simulink model "emr_library_custom"  (R2025b)
settings: Solver=ode45  StartTime=0.0  StopTime=10.0  RelTol=1e-3  EnableMultiTasking=on
settings Model: ExtModeTrigMode=oneshot  ExtModeArmWhenConnect=off  Creator=Tony  LastModifiedBy=opatiny
settings SolverCC: AlgebraicLoopSolver=TrustRegion
settings DataIOCC: SaveFormat=Array  SignalLoggingSaveFormat=ModelDataLogs  ReturnWorkspaceOutputs=off  SignalLoggingName=sigsOut
settings OptimizationCC: BooleanDataType=off  ExpressionDepthLimit=2147483647.0  LifeSpan=inf
settings DebuggingCC: SaveWithParameterizedLinksMsg=none  UnderspecifiedInitializationDetection=Classic  MergeDetectMultiDrivingBlocksExec=none  SignalResolutionControl=TryResolveAllWithWarning  MultiTaskDSMMsg=warning  MultiTaskCondExecSysMsg=none  FcnCallInpInsideContextMsg=warning  UnconnectedInputMsg=warning  UnconnectedOutputMsg=warning  UnconnectedLineMsg=warning  StateNameClashWarn=warning  SFUnexpectedBacktrackingDiag=warning  SFNoUnconditionalDefaultTransitionDiag=warning  SFExecutionAtInitializationDiag=none  ArithmeticOperatorsInVariantConditions=warning
settings HardwareCC: ProdBitPerPointer=32.0  ProdBitPerSizeT=32.0  ProdBitPerPtrDiffT=32.0  ProdLargestAtomicFloat=None  ProdIntDivRoundTo=Undefined  ProdEndianess=Unspecified  ProdWordSize=32.0  ProdHWDeviceType=32-bit Generic  TargetUnknown=on
settings ModelReferenceCC: PropagateSignalLabelsOutOfModel=off
settings SFSimCC: SimUseLocalCustomCode=off  CustomCodeUndefinedFunction=UseInterfaceOnly
settings RTWCC: RTWUseLocalCustomCode=off  GPUComputeCapability=3.5
settings CodeAppCC: StateflowObjectComments=on
settings GRTTargetCC: TargetLangStandard=C89/C90 (ANSI)  CombineOutputUpdateFcns=off  GRTInterface=on
settings ConfigComp: CovMetricSettings=dw  CovSaveCumulativeToWorkspaceVar=on  CovSaveSingleToWorkspaceVar=on  CovExternalEMLEnable=off  CovSFcnEnable=off

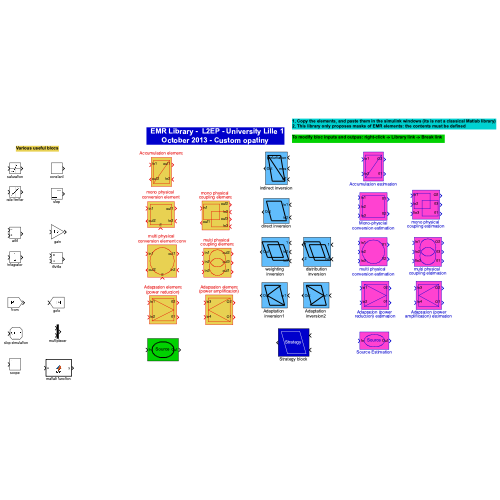
[thumbnail: Simulink's stored preview of the top-level diagram]
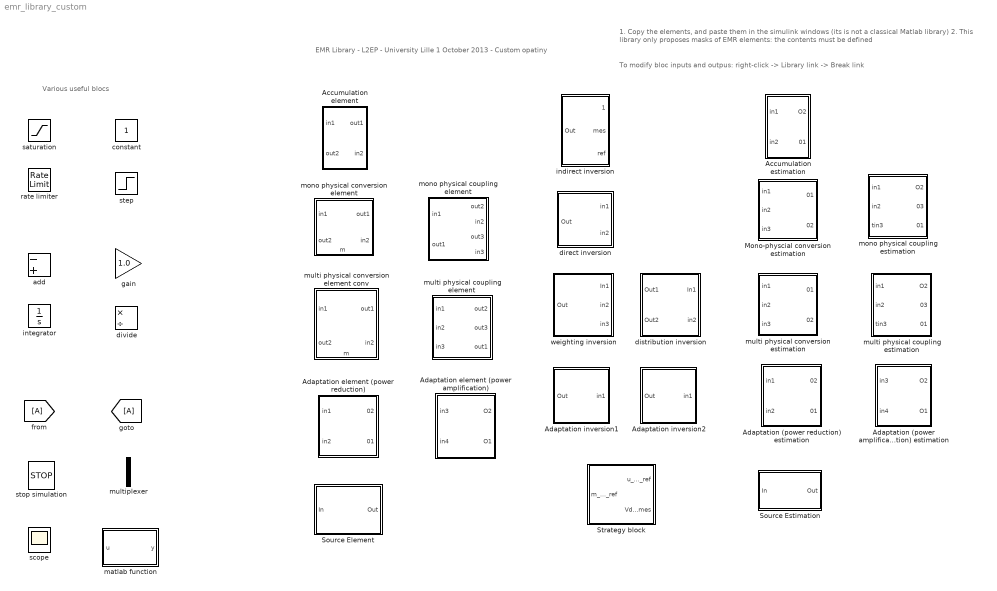
== system emr_library_custom ==
  note: EMR Library -  L2EP - University Lille 1
      | October 2013 - Custom opatiny
  note: 1. Copy the elements, and paste them in the simulink windows (its is not a classical Matlab library)
      | 2. This library only proposes masks of EMR elements: the contents must be defined
  note: Various useful blocs
  note: To modify bloc inputs and outpus: right-click -> Library link -> Break link
  Accumulation element : Subsystem  mask(CM){}
      settings: PortSchema="{\"entries\":[{\"content\":{\"sides\":[{\"content\":{\"connectorIds\":[\"In1\",\"Out2\"]},\"type\":\"ConnectorPlacement.EquallySpacedRectSide\",\"uuid\":\"ce6d3bac-983c-4cc2-8cf0-29bd76c88970\"},{\"content\":{\"connectorIds\":[\"Out1\",\"In2\"],\"side\":\"RIGHT\"},\"type\":\"ConnectorPlacement.EquallySpacedRectSide\",\"uuid\":\"5515666e-487b-4d04-97a1-137c298a6b81\"},{\"content\":{\"side\":\"TOP\"},\"type\":\"ConnectorPlacement.EquallySpacedRectSide\",\"uuid\":\"e218289f-4799-4b6c-b17f-c7c3909bc728\"}]},\"type\":\"ConnectorPlacement.EquallySpacedConnector\",\"uuid\":\"8de20a8e-e66a-466f-89a2-5b2e75b7ec3a\"}],\"packageUris\":[\"http://schema.mathworks.com/mf0/Connector/R2020b\"],\"version\":\"1.0\"}"
      mask Display: plot(0,0,100,100,[10,10,90,90,10],[90,10,10,90,90], [10,90],[10,90])
  Accumulation estimation : Subsystem  AncestorBlock=simulink/REM/EA  mask(CM){}
      mask Display: plot(0,0,100,100,[10,10,90,90,10],[90,10,10,90,90], [10,90],[10,90])
  Adaptation inversion1 : Subsystem  AncestorBlock=simulink/SMC/Inversion EC avec mesure
      mask Display: plot(0,0,100,100, [10,30,90,70,10],[90,10,10,90,90], [90,20,75],[10,50,90])
  Adaptation inversion2 : Subsystem  AncestorBlock=simulink/SMC/Inversion EC avec mesure
      mask Display: plot(0,0,100,100, [10,30,90,70,10],[90,10,10,90,90], [25,80,10],[10,50,90])
  Adaptation (power amplification) estimation : Subsystem  AncestorBlock=simulink/REM/EA  mask(CM){}
      mask Display: plot(0,0,100,100, [10,10,90,90,10],[90,10,10,90,90], [90,10,90],[10,50,90])
  Adaptation (power reduction) estimation : Subsystem  AncestorBlock=simulink/REM/EA  mask(CM){}
      mask Display: plot(0,0,100,100, [10,10,90,90,10],[90,10,10,90,90], [10,90,10],[10,50,90])
  Adaptation element (power amplification) : Subsystem  AncestorBlock=simulink/REM/EA  mask(CM){}
      mask Display: plot(0,0,100,100, [10,10,90,90,10],[90,10,10,90,90], [90,10,90],[10,50,90])
  Adaptation element (power reduction) : Subsystem  mask(CM){}
      mask Display: plot(0,0,100,100, [10,10,90,90,10],[90,10,10,90,90], [10,90,10],[10,50,90])
  Mono-physcial conversion estimation : Subsystem  AncestorBlock=simulink/REM/EC Elec  mask(Hacheur){}
      mask Display: plot(0,0,100,100,[10,10,90,90,10],[90,10,10,90,90])
  Source Element : Subsystem  AncestorBlock=simulink/REM/SE
      mask Display:
      | plot(0,0,100,100, 1.2*[50,57.68,60.77,63.08,64.97,66.58,68,69.26,70.4, 	71.42,72.36,78.28,80,78.28,72.36,71.42,70.4, 	69.26,68,66.58,64.97,63.08,60.77,57.68,50,42.32, 	39.23,36.92,35.03,33.42,32,30.74,29.6,28.58, 	27.64,21.72,20,21.72,27.64,28.58,29.6,30.74,32, 	33.42,35.03,36.92,39.23,42.32,50]-10, 1.2*[20,21,22,23,24,25,26,27,28,29,30,40,50,60,70,71,72, 	73,74,75,76,77,78,79,80,79,78,77,76,75,74,73,72, 	71,70,60,50,40,30,29,28,27,26,25,24,23,22,21,20]-10)
      | disp('Source')
  Source Estimation : Subsystem  AncestorBlock=simulink/REM/SE
      mask Display:
      | plot(0,0,100,100, 1.2*[50,57.68,60.77,63.08,64.97,66.58,68,69.26,70.4, 	71.42,72.36,78.28,80,78.28,72.36,71.42,70.4, 	69.26,68,66.58,64.97,63.08,60.77,57.68,50,42.32, 	39.23,36.92,35.03,33.42,32,30.74,29.6,28.58, 	27.64,21.72,20,21.72,27.64,28.58,29.6,30.74,32, 	33.42,35.03,36.92,39.23,42.32,50]-10, 1.2*[20,21,22,23,24,25,26,27,28,29,30,40,50,60,70,71,72, 	73,74,75,76,77,78,79,80,79,78,77,76,75,74,73,72, 	71,70,60,50,40,30,29,28,27,26,25,24,23,22,21,20]-10)
      | disp('Source')
  Strategy block : Subsystem  AncestorBlock=simulink/SMC/Inversion EC avec mesure
      mask Display:
      | color('white')
      | plot(0,0,100,100,[10,30,90,70,10],[90,10,10,90,90])
      | disp('Strategy')
  add : Sum  Inputs=-+
  constant : Constant
  direct inversion : Subsystem  AncestorBlock=simulink/SMC/Inversion EC avec mesure
      mask Display: plot(0,0,100,100,[10,30,90,70,10],[90,10,10,90,90])
  distribution inversion : Subsystem  AncestorBlock=simulink/SMC/Bloc de répartition
      mask Display: plot(0,0,100,100,[20,40,100,80,20],[75,20,20,75,75], [0,20,80,60,0],[85,30,30,85,85])
  divide : Product  Inputs=*/
  from : From
  gain : Gain  Gain=1.0
  goto : Goto
  indirect inversion : Subsystem  AncestorBlock=simulink/SMC/Asservissement Correcteur IP
      mask Display: plot(0,0,100,100, [10,30,90,70,10,90],[90,10,10,90,90,10])
  integrator : Integrator
  matlab function : MATLAB Function  TreatAsAtomicUnit=on
  mono physical conversion element : Subsystem  mask(Hacheur){}
      settings: PortSchema="{\"entries\":[{\"content\":{\"sides\":[{\"content\":{\"connectorIds\":[\"In1\",\"Out2\"]},\"type\":\"ConnectorPlacement.EquallySpacedRectSide\",\"uuid\":\"62d3361f-f49a-4a89-b7fa-c77fcee42868\"},{\"content\":{\"connectorIds\":[\"Out1\",\"In3\"],\"side\":\"RIGHT\"},\"type\":\"ConnectorPlacement.EquallySpacedRectSide\",\"uuid\":\"da99363c-611b-4582-b369-34120805217f\"},{\"content\":{\"side\":\"TOP\"},\"type\":\"ConnectorPlacement.EquallySpacedRectSide\",\"uuid\":\"7aa74fda-98a3-42bb-9007-2e39de70bf34\"},{\"content\":{\"connectorIds\":[\"In2\"],\"side\":\"BOTTOM\"},\"type\":\"ConnectorPlacement.EquallySpacedRectSide\",\"uuid\":\"47df5eac-c768-4899-b572-df26d6841fea\"}]},\"type\":\"ConnectorPlacement.EquallySpacedConnector\",\"uuid\":\"6baec6e9-7443-4760-93d1-cc70873952bd\"}],\"packageUris\":[\"http://schema.mathworks.com/mf0/Connector/R2020b\"],\"version\":\"1.0\"}"
      mask Display: plot(0,0,100,100,[10,10,90,90,10],[90,10,10,90,90])
  mono physical coupling element : Subsystem  mask(CM){}
      settings: PortSchema="{\"entries\":[{\"content\":{\"sides\":[{\"content\":{\"connectorIds\":[\"In1\",\"Out3\"]},\"type\":\"ConnectorPlacement.EquallySpacedRectSide\",\"uuid\":\"a0cc6eb3-0f35-4a31-afc0-a3cae9b9d5bb\"},{\"content\":{\"connectorIds\":[\"Out1\",\"In2\",\"Out2\",\"In3\"],\"side\":\"RIGHT\"},\"type\":\"ConnectorPlacement.EquallySpacedRectSide\",\"uuid\":\"f0fc86c1-6f18-402b-9eea-d081ace87e62\"},{\"content\":{\"connectorIds\":[],\"side\":\"TOP\"},\"type\":\"ConnectorPlacement.EquallySpacedRectSide\",\"uuid\":\"dfd8824c-ea43-4486-a7b0-05621e67d875\"}]},\"type\":\"ConnectorPlacement.EquallySpacedConnector\",\"uuid\":\"18c849d2-2a12-4239-b86e-b7a06eec8617\"}],\"packageUris\":[\"http://schema.mathworks.com/mf0/Connector/R2020b\"],\"version\":\"1.0\"}"
      mask Display: plot(0,0,100,100,[35,35,95,95,35],[65,10,10,65,65], [5,5,65,65,5],[90,35,35,90,90])
  mono physical coupling estimation : Subsystem  mask(CM){}
      mask Display: plot(0,0,100,100,[35,35,95,95,35],[65,10,10,65,65], [5,5,65,65,5],[90,35,35,90,90])
  multi physical conversion element conv : Subsystem
      settings: PortSchema="{\"entries\":[{\"content\":{\"sides\":[{\"content\":{\"connectorIds\":[\"In1\",\"Out2\"]},\"type\":\"ConnectorPlacement.EquallySpacedRectSide\",\"uuid\":\"61fbc010-38ff-4a80-98f4-f5d8a9e77fd8\"},{\"content\":{\"connectorIds\":[\"Out1\",\"In3\"],\"side\":\"RIGHT\"},\"type\":\"ConnectorPlacement.EquallySpacedRectSide\",\"uuid\":\"7ae9e15d-ee0f-4ba6-b3b7-5dcbca441e0a\"},{\"content\":{\"connectorIds\":[],\"side\":\"TOP\"},\"type\":\"ConnectorPlacement.EquallySpacedRectSide\",\"uuid\":\"f4fbe656-3ef3-486e-b25e-f340040f3905\"},{\"content\":{\"connectorIds\":[\"In2\"],\"side\":\"BOTTOM\"},\"type\":\"ConnectorPlacement.EquallySpacedRectSide\",\"uuid\":\"742d13fb-c4a1-4c94-b7a0-3eefa6669287\"}]},\"type\":\"ConnectorPlacement.EquallySpacedConnector\",\"uuid\":\"024d92c1-e2c4-4b69-9482-c403c9d240aa\"}],\"packageUris\":[\"http://schema.mathworks.com/mf0/Connector/R2020b\"],\"version\":\"1.0\"}"
      mask Display: plot(0,0,100,100, 1.4*[50,57.68,60.77,63.08,64.97,66.58,68,69.26,70.4, 	71.42,72.36,78.28,80,78.28,72.36,71.42,70.4, 	69.26,68,66.58,64.97,63.08,60.77,57.68,50,42.32, 	39.23,36.92,35.03,33.42,32,30.74,29.6,28.58, 	27.64,21.72,20,21.72,27.64,28.58,29.6,30.74,32, 	33.42,35.03,36.92,39.23,42.32,50]-20, 1.4*[20,21,22,23,24,25,26,27,28,29,30,40,50,60,70,71,72, 	73,74,75,76,77,78,79,80,79,78,77,76,75,74,73,72, 	71,70,60,50,40,30,29,28,27,26,25,24,23,22,21,20]-20)
  multi physical conversion estimation : Subsystem  AncestorBlock=simulink/REM/EC EM
      mask Display: plot(0,0,100,100, 1.4*[50,57.68,60.77,63.08,64.97,66.58,68,69.26,70.4, 	71.42,72.36,78.28,80,78.28,72.36,71.42,70.4, 	69.26,68,66.58,64.97,63.08,60.77,57.68,50,42.32, 	39.23,36.92,35.03,33.42,32,30.74,29.6,28.58, 	27.64,21.72,20,21.72,27.64,28.58,29.6,30.74,32, 	33.42,35.03,36.92,39.23,42.32,50]-20, 1.4*[20,21,22,23,24,25,26,27,28,29,30,40,50,60,70,71,72, 	73,74,75,76,77,78,79,80,79,78,77,76,75,74,73,72, 	71,70,60,50,40,30,29,28,27,26,25,24,23,22,21,20]-20)
  multi physical coupling element : Subsystem  mask(CM){}
      mask Display: plot(0,0,100,100, [50,57.68,60.77,63.08,64.97,66.58,68,69.26,70.4, 	71.42,72.36,78.28,80,78.28,72.36,71.42,70.4, 	69.26,68,66.58,64.97,63.08,60.77,57.68,50,42.32, 	39.23,36.92,35.03,33.42,32,30.74,29.6,28.58, 	27.64,21.72,20,21.72,27.64,28.58,29.6,30.74,32, 	33.42,35.03,36.92,39.23,42.32,50], [20,21,22,23,24,25,26,27,28,29,30,40,50,60,70,71,72, 	73,74,75,76,77,78,79,80,79,78,77,76,75,74,73,72, 	71,70,60,50,40,30,29,28,27,26,25,24,23,22,21,20]-15,  [50,57.68,60.77,63.08,64.97,66.58,68,69.26,70.4, 	71.42,72.36,78.28,80,78.28,72.36,71.42,70.4, 	69.26,68,66.58,64.97,63.08,60.77,57.68,50,42.32, 	39.23,36.92,35.03,33.42,32,30.74,29.6,28.58, 	27.64,21.72,20,21.72,27.64,28.58,29.6,30.74,32, 	33.42,35.03,36.92,39.23,42.32,50], [20,21,22,23,24,25,26,27,28,29,30,40,50,60,70,71,72, 	73,74,75,76,77,78,79,80,79,78,77,76,75,74,73,72, 	71,70,60,50,40,30,29,28,27,26,25,24,23,22,21,20]+15)
  multi physical coupling estimation : Subsystem  mask(CM){}
      mask Display: plot(0,0,100,100, [50,57.68,60.77,63.08,64.97,66.58,68,69.26,70.4, 	71.42,72.36,78.28,80,78.28,72.36,71.42,70.4, 	69.26,68,66.58,64.97,63.08,60.77,57.68,50,42.32, 	39.23,36.92,35.03,33.42,32,30.74,29.6,28.58, 	27.64,21.72,20,21.72,27.64,28.58,29.6,30.74,32, 	33.42,35.03,36.92,39.23,42.32,50], [20,21,22,23,24,25,26,27,28,29,30,40,50,60,70,71,72, 	73,74,75,76,77,78,79,80,79,78,77,76,75,74,73,72, 	71,70,60,50,40,30,29,28,27,26,25,24,23,22,21,20]-15,  [50,57.68,60.77,63.08,64.97,66.58,68,69.26,70.4, 	71.42,72.36,78.28,80,78.28,72.36,71.42,70.4, 	69.26,68,66.58,64.97,63.08,60.77,57.68,50,42.32, 	39.23,36.92,35.03,33.42,32,30.74,29.6,28.58, 	27.64,21.72,20,21.72,27.64,28.58,29.6,30.74,32, 	33.42,35.03,36.92,39.23,42.32,50], [20,21,22,23,24,25,26,27,28,29,30,40,50,60,70,71,72, 	73,74,75,76,77,78,79,80,79,78,77,76,75,74,73,72, 	71,70,60,50,40,30,29,28,27,26,25,24,23,22,21,20]+15)
  multiplexer : Mux  Inputs=2
  rate limiter : RateLimiter  SampleTimeMode=inherited
  saturation : Saturate
  scope : Scope
  step : Step  SampleTime=0
  stop simulation : Stop
  weighting inversion : Subsystem  AncestorBlock=simulink/SMC/Bloc de pondération
      mask Display: plot(0,0,100,100,[20,40,100,80,20],[75,20,20,75,75], [0,20,80,60,0],[85,30,30,85,85])

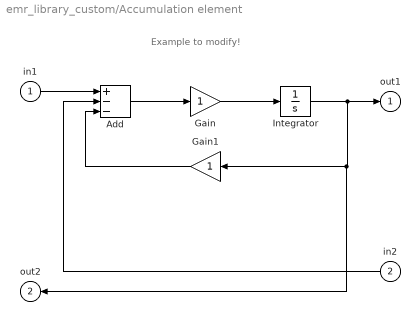
== system emr_library_custom/Accumulation element ==
  note: Example to modify!
  in1 : Inport
  in2 : Inport  Port=2
  Add : Sum  Inputs=+--
  Gain : Gain
  Gain1 : Gain
  Integrator : Integrator
  out1 : Outport  InitialOutput=0
  out2 : Outport  Port=2  InitialOutput=0
  wires:
  Add/1 -> Gain/1
  in1/1 -> Add/1
  Integrator/1 -> out1/1, out2/1, Gain1/1
  in2/1 -> Add/2
  Gain/1 -> Integrator/1
  Gain1/1 -> Add/3

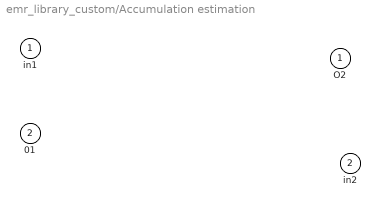
== system emr_library_custom/Accumulation estimation ==
  in1 : Inport
  in2 : Inport  Port=2
  O2 : Outport  InitialOutput=0
  01 : Outport  Port=2  InitialOutput=0

== system emr_library_custom/Adaptation inversion1 ==
  in1 : Inport
  Out : Outport  InitialOutput=0

== system emr_library_custom/Adaptation inversion2 ==
  in1 : Inport
  Out : Outport  InitialOutput=0

== system emr_library_custom/Adaptation (power amplification) estimation ==
  in3 : Inport
  in4 : Inport  Port=2
  O2 : Outport  InitialOutput=0
  O1 : Outport  Port=2  InitialOutput=0

== system emr_library_custom/Adaptation (power reduction) estimation ==
  in1 : Inport
  in2 : Inport  Port=2
  02 : Outport  InitialOutput=0
  01 : Outport  Port=2  InitialOutput=0

== system emr_library_custom/Adaptation element (power amplification) ==
  in3 : Inport
  in4 : Inport  Port=2
  O2 : Outport  InitialOutput=0
  O1 : Outport  Port=2  InitialOutput=0

== system emr_library_custom/Adaptation element (power reduction) ==
  in1 : Inport
  in2 : Inport  Port=2
  02 : Outport  InitialOutput=0
  01 : Outport  Port=2  InitialOutput=0

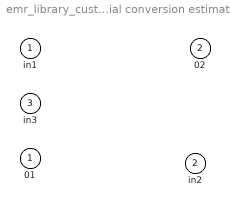
== system emr_library_custom/Mono-physcial conversion estimation ==
  in1 : Inport
  in2 : Inport  Port=2
  in3 : Inport  Port=3
  01 : Outport  InitialOutput=0
  02 : Outport  Port=2  InitialOutput=0

== system emr_library_custom/Source Element ==
  In : Inport
  Out : Outport  InitialOutput=0

== system emr_library_custom/Source Estimation ==
  In : Inport
  Out : Outport  InitialOutput=0

== system emr_library_custom/Strategy block ==
  u_hind_ref : Inport
  Vdc_mes : Inport  Port=2
  m_hind_ref : Outport  InitialOutput=0

== system emr_library_custom/direct inversion ==
  in1 : Inport
  in2 : Inport  Port=2
  Out : Outport  InitialOutput=0

== system emr_library_custom/distribution inversion ==
  In1 : Inport
  in2 : Inport  Port=2
  Out1 : Outport  InitialOutput=0
  Out2 : Outport  Port=2  InitialOutput=0

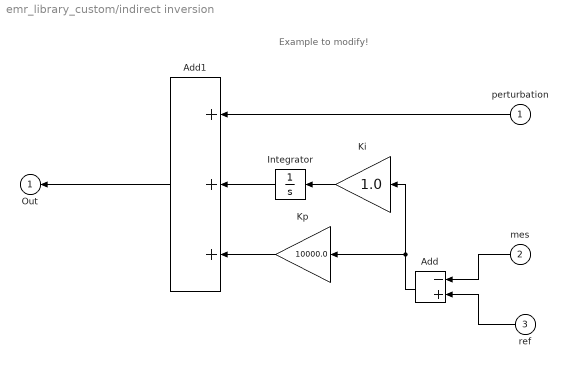
== system emr_library_custom/indirect inversion ==
  note: Example to modify!
  perturbation : Inport
  mes : Inport  Port=2
  ref : Inport  Port=3
  Add : Sum  Inputs=-+
  Add1 : Sum  Inputs=+++
  Integrator : Integrator
  Ki : Gain  Gain=1.0
  Kp : Gain  Gain=10000.0
  Out : Outport  InitialOutput=0
  wires:
  perturbation/1 -> Add1/1
  Add/1 -> Ki/1, Kp/1
  Kp/1 -> Add1/3
  Add1/1 -> Out/1
  mes/1 -> Add/1
  Integrator/1 -> Add1/2
  Ki/1 -> Integrator/1
  ref/1 -> Add/2

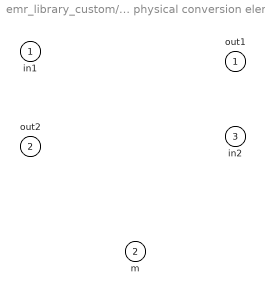
== system emr_library_custom/mono physical conversion element ==
  in1 : Inport
  m : Inport  Port=2
  in2 : Inport  Port=3
  out1 : Outport  InitialOutput=0
  out2 : Outport  Port=2  InitialOutput=0

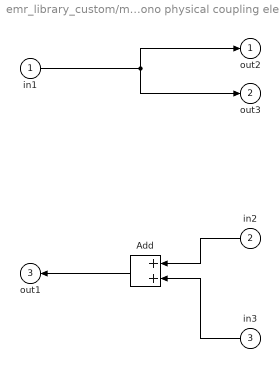
== system emr_library_custom/mono physical coupling element ==
  in1 : Inport
  in2 : Inport  Port=2
  in3 : Inport  Port=3
  Add : Sum
  out2 : Outport  InitialOutput=0  VectorParamsAs1DForOutWhenUnconnected=off
  out3 : Outport  Port=2  InitialOutput=0  VectorParamsAs1DForOutWhenUnconnected=off
  out1 : Outport  Port=3  InitialOutput=0  VectorParamsAs1DForOutWhenUnconnected=off
  wires:
  in1/1 -> out3/1, out2/1
  in2/1 -> Add/1
  in3/1 -> Add/2
  Add/1 -> out1/1

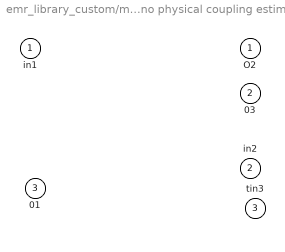
== system emr_library_custom/mono physical coupling estimation ==
  in1 : Inport
  in2 : Inport  Port=2
  tin3 : Inport  Port=3
  O2 : Outport  InitialOutput=0
  03 : Outport  Port=2  InitialOutput=0
  01 : Outport  Port=3  InitialOutput=0

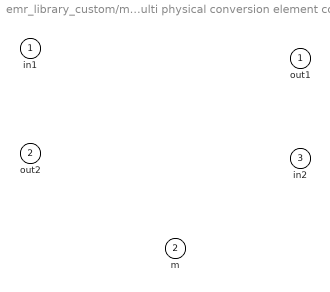
== system emr_library_custom/multi physical conversion element conv ==
  in1 : Inport
  m : Inport  Port=2
  in2 : Inport  Port=3
  out1 : Outport  InitialOutput=0
  out2 : Outport  Port=2  InitialOutput=0

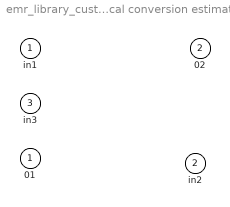
== system emr_library_custom/multi physical conversion estimation ==
  in1 : Inport
  in2 : Inport  Port=2
  in3 : Inport  Port=3
  01 : Outport  InitialOutput=0
  02 : Outport  Port=2  InitialOutput=0

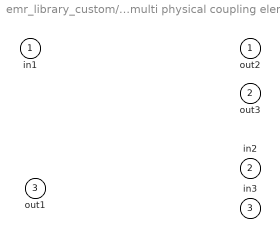
== system emr_library_custom/multi physical coupling element ==
  in1 : Inport
  in2 : Inport  Port=2
  in3 : Inport  Port=3
  out2 : Outport  InitialOutput=0
  out3 : Outport  Port=2  InitialOutput=0
  out1 : Outport  Port=3  InitialOutput=0

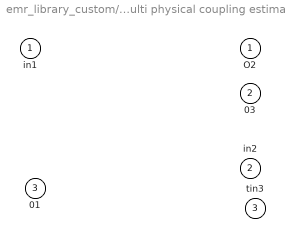
== system emr_library_custom/multi physical coupling estimation ==
  in1 : Inport
  in2 : Inport  Port=2
  tin3 : Inport  Port=3
  O2 : Outport  InitialOutput=0
  03 : Outport  Port=2  InitialOutput=0
  01 : Outport  Port=3  InitialOutput=0

== system emr_library_custom/weighting inversion ==
  In1 : Inport
  in2 : Inport  Port=2
  in3 : Inport  Port=3
  Out : Outport  InitialOutput=0

== matlab function emr_library_custom/matlab function ==
  data: u input; y output
function y = fcn(u)

y = u;
